simulink model "example_of_convert_voltage_to_current_and_vise_verse"  (R2021a)
settings: Solver=VariableStepAuto  StartTime=0.0  StopTime=10.0  RelTol=1e-3
settings Model: Creator=YasserNet  LastModifiedBy=YasserNet

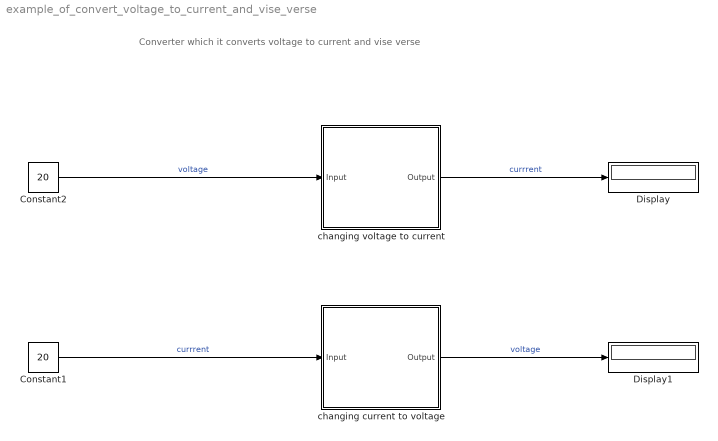
== system example_of_convert_voltage_to_current_and_vise_verse ==
  note: Converter which it converts voltage to current and vise verse
  Constant1 : Constant  Value=20
  Constant2 : Constant  Value=20
  Display : Display
  Display1 : Display
  changing current to voltage : Subsystem
  "changing voltage to current " : Subsystem
  wires:
  "changing voltage to current "/1(Output) -> Display/1  "currrent"
  Constant2/1 -> "changing voltage to current "/1(Input)  "voltage"
  Constant1/1 -> changing current to voltage/1(Input)  "currrent"
  changing current to voltage/1(Output) -> Display1/1  "voltage"

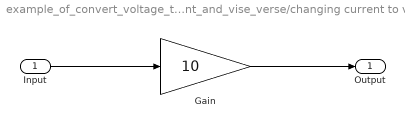
== system example_of_convert_voltage_to_current_and_vise_verse/changing current to voltage ==
  Input : Inport
  Gain : Gain  Gain=10
  Output : Outport
  wires:
  Input/1 -> Gain/1
  Gain/1 -> Output/1

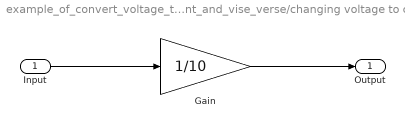
== system example_of_convert_voltage_to_current_and_vise_verse/changing voltage to current  ==
  Input : Inport
  Gain : Gain  Gain=1/10
  Output : Outport
  wires:
  Input/1 -> Gain/1
  Gain/1 -> Output/1
